simulink model "heaveCompMichael_v03_tollax_spesial"  (R2021b)
settings: Solver=VariableStepAuto  StartTime=0.0  StopTime=50  RelTol=1e-3
model workspace (MATLAB code in the model file):
  | %fluid data
  | rho = 875;
  | %valve config
  | P_r = 70e5;
  | Cd = 0.7;
  | Q_r = 200/6e4;
  | AdMax = Q_r/Cd/sqrt(2/rho*P_r/2);
  | 
  | g = 9.81;                   %gravity
  | zw = 0.8;                   %wave amplitude
  | tw = 10;                    %total wave period
  | ig = 46;                    %gear ratio gearbox
  | m = 9000;                   %mass of payload
  | mueq = 0.15;                %friction coeffisient
  | dd = 0.45;                  %diameter drum
  | nyv = 0.92;                 %volumetric effissiency
  | rd = dd/2;                  %radius drum
  | omega0 = 5;                 %velosity in friction equation
  | omegap = 1500;              %velosity hpu pump
  | nsh = 3;
  | gearrationsh = nsh.*2;
libraries: fl_lib x18, nesl_utility x11, sh_lib x4, slpidlib x1
settings Model: Creator=tolla  LastModifiedBy=marcu

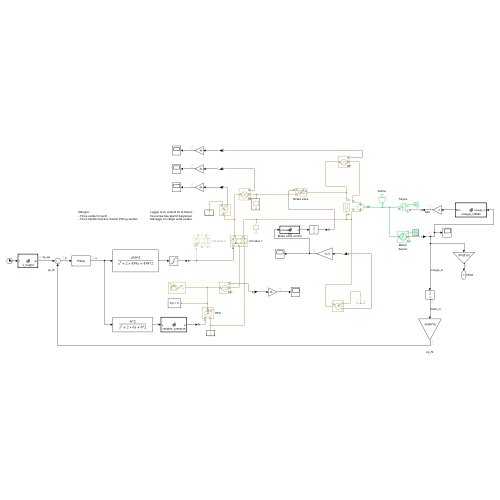
[thumbnail: Simulink's stored preview of the top-level diagram]
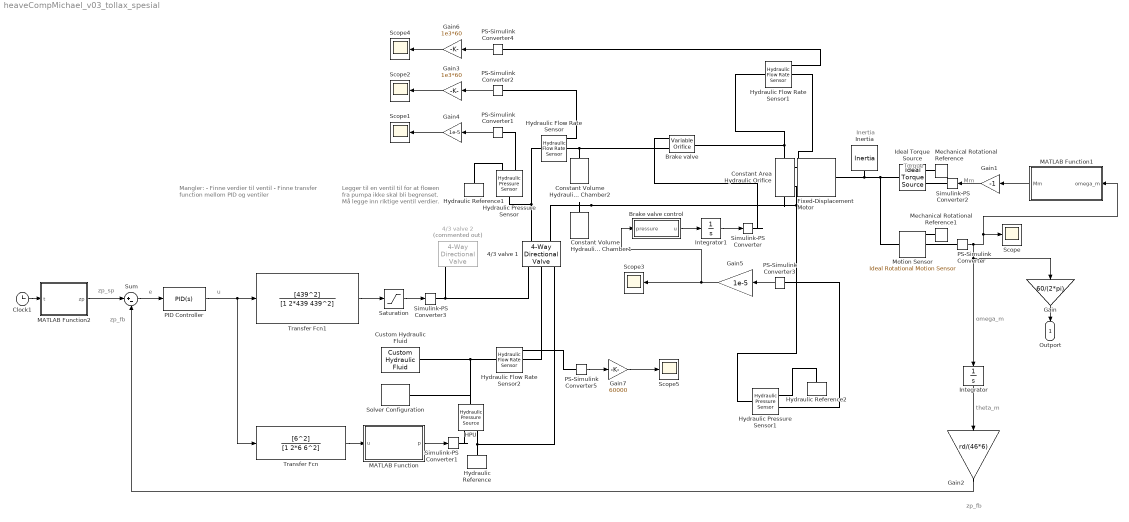
== system heaveCompMichael_v03_tollax_spesial ==
  note: Mangler:
      | - Finne verdier til ventil
      | - Finne transfer function mellom PID og ventiler
  note: Mm
  note: Legger til en ventil til for at flowen
      | fra pumpa ikke skal bli begrenset.
      | Må legge inn riktige ventil verdier.
  note: e
  note: u
  note: zp_fb
  note: zp_sp
  note: zp_fb
  note: theta_m
  note: omega_m
  note: Torque
  note: Inertia
  4/3 valve 1 : sh_lib/Valves/Directional Valves/4-Way Directional Valve  area_spec=sh.valves.directional_valves.enum.area_spec.identical  mdl_type_identical=sh.valves.directional_valves.enum.mdl_type.linear  mdl_type_different=sh.valves.directional_valves.enum.mdl_type.linear  interp_method_identical=sh.valves.directional_valves.enum.interp_method.linear  interp_method_different=sh.valves.directional_valves.enum.interp_method.linear  extrap_method_identical=sh.valves.directional_valves.enum.extrap_method.linear  extrap_method_different=sh.valves.directional_valves.enum.extrap_method.linear  A_leak=1e-12 m^2  C_d=Cd  lam_spec=sh.valves.directional_valves.enum.lam_spec.pressure_ratio  B_lam=0.999  Re_cr=12  opening_max=1 m  area_max=3.7646e-5 m^2  opening_max_P_A=0.005 m  area_max_P_A=0.5e-4 m^2  opening_max_P_B=0.005 m  area_max_P_B=0.5e-4 m^2  opening_max_A_T=0.005 m  area_max_A_T=0.5e-4 m^2  opening_max_B_T=0.005 m  area_max_B_T=0.5e-4 m^2  opening_area_tab=[-.002, 0, .002, .005, .015] m  area_tab=[1e-09, 2.0352e-07, 4.0736e-05, .00011438, .00034356] m^2  opening_flow_rate_tab=[-.002, 0, .002, .005, .015] m  pressure_tab=[-10000000, -5000000, -2000000, 2000000, 5000000, 10000000] Pa  flow_rate_tab=[-1e-07, -7.0711e-08, -4.4721e-08, 4.4721e-08, 7.0711e-08, 1e-07; -2.0352e-05, -1.4391e-05, -9.1017e-06, 9.1017e-06, 1.4391e-05, 2.0352e-05; -.0040736, -.0028805, -.0018218, .0018218, .0028805, .0040736; -.011438, -.0080879, -.0051152, .0051152, .0080879, .011438; -.034356, -.024293, -.015364, .015364, .024293, .034356] m^3/s  opening_area_tab_P_A=[-.002, 0, .002, .005, .015] m  area_tab_P_A=[1e-09, 2.0352e-07, 4.0736e-05, .00011438, .00034356] m^2  opening_flow_rate_tab_P_A=[-.002, 0, .002, .005, .015] m  pressure_tab_P_A=[-10000000, -5000000, -2000000, 2000000, 5000000, 10000000] Pa  flow_rate_tab_P_A=[-1e-07, -7.0711e-08, -4.4721e-08, 4.4721e-08, 7.0711e-08, 1e-07; -2.0352e-05, -1.4391e-05, -9.1017e-06, 9.1017e-06, 1.4391e-05, 2.0352e-05; -.0040736, -.0028805, -.0018218, .0018218, .0028805, .0040736; -.011438, -.0080879, -.0051152, .0051152, .0080879, .011438; -.034356, -.024293, -.015364, .015364, .024293, .034356] m^3/s  opening_area_tab_P_B=[-.002, 0, .002, .005, .015] m  area_tab_P_B=[1e-09, 2.0352e-07, 4.0736e-05, .00011438, .00034356] m^2  opening_flow_rate_tab_P_B=[-.002, 0, .002, .005, .015] m  pressure_tab_P_B=[-10000000, -5000000, -2000000, 2000000, 5000000, 10000000] Pa  flow_rate_tab_P_B=[-1e-07, -7.0711e-08, -4.4721e-08, 4.4721e-08, 7.0711e-08, 1e-07; -2.0352e-05, -1.4391e-05, -9.1017e-06, 9.1017e-06, 1.4391e-05, 2.0352e-05; -.0040736, -.0028805, -.0018218, .0018218, .0028805, .0040736; -.011438, -.0080879, -.0051152, .0051152, .0080879, .011438; -.034356, -.024293, -.015364, .015364, .024293, .034356] m^3/s  opening_area_tab_A_T=[-.002, 0, .002, .005, .015] m  area_tab_A_T=[1e-09, 2.0352e-07, 4.0736e-05, .00011438, .00034356] m^2  opening_flow_rate_tab_A_T=[-.002, 0, .002, .005, .015] m  pressure_tab_A_T=[-10000000, -5000000, -2000000, 2000000, 5000000, 10000000] Pa  flow_rate_tab_A_T=[-1e-07, -7.0711e-08, -4.4721e-08, 4.4721e-08, 7.0711e-08, 1e-07; -2.0352e-05, -1.4391e-05, -9.1017e-06, 9.1017e-06, 1.4391e-05, 2.0352e-05; -.0040736, -.0028805, -.0018218, .0018218, .0028805, .0040736; -.011438, -.0080879, -.0051152, .0051152, .0080879, .011438; -.034356, -.024293, -.015364, .015364, .024293, .034356] m^3/s  opening_area_tab_B_T=[-.002, 0, .002, .005, .015] m  area_tab_B_T=[1e-09, 2.0352e-07, 4.0736e-05, .00011438, .00034356] m^2  opening_flow_rate_tab_B_T=[-.002, 0, .002, .005, .015] m  pressure_tab_B_T=[-10000000, -5000000, -2000000, 2000000, 5000000, 10000000] Pa  flow_rate_tab_B_T=[-1e-07, -7.0711e-08, -4.4721e-08, 4.4721e-08, 7.0711e-08, 1e-07; -2.0352e-05, -1.4391e-05, -9.1017e-06, 9.1017e-06, 1.4391e-05, 2.0352e-05; -.0040736, -.0028805, -.0018218, .0018218, .0028805, .0040736; -.011438, -.0080879, -.0051152, .0051152, .0080879, .011438; -.034356, -.024293, -.015364, .015364, .024293, .034356] m^3/s  x_0_P_A=0 m  x_0_P_B=0 m  x_0_A_T=0 m  x_0_B_T=0 m
      settings: InternalSimscapePortConfiguration="{\"Bottom\":[],\"Left\":[{\"id\":\"A\",\"label\":\"A\",\"type\":\"foundation.hydraulic.hydraulic\"},{\"id\":\"B\",\"label\":\"B\",\"type\":\"foundation.hydraulic.hydraulic\"}],\"Right\":[{\"id\":\"S\",\"label\":\"S\",\"type\":\"input\"},{\"id\":\"P\",\"label\":\"P\",\"type\":\"foundation.hydraulic.hydraulic\"},{\"id\":\"T\",\"label\":\"T\",\"type\":\"foundation.hydraulic.hydraulic\"}],\"Top\":[]}"
  4/3 valve 2 : sh_lib/Valves/Directional Valves/4-Way Directional Valve  Commented=on  area_spec=sh.valves.directional_valves.enum.area_spec.identical  mdl_type_identical=sh.valves.directional_valves.enum.mdl_type.linear  mdl_type_different=sh.valves.directional_valves.enum.mdl_type.linear  interp_method_identical=sh.valves.directional_valves.enum.interp_method.linear  interp_method_different=sh.valves.directional_valves.enum.interp_method.linear  extrap_method_identical=sh.valves.directional_valves.enum.extrap_method.linear  extrap_method_different=sh.valves.directional_valves.enum.extrap_method.linear  A_leak=1e-12 m^2  C_d=Cd  lam_spec=sh.valves.directional_valves.enum.lam_spec.pressure_ratio  B_lam=0.999  Re_cr=12  opening_max=1 m  area_max=3.7646e-5 m^2  opening_max_P_A=0.005 m  area_max_P_A=0.5e-4 m^2  opening_max_P_B=0.005 m  area_max_P_B=0.5e-4 m^2  opening_max_A_T=0.005 m  area_max_A_T=0.5e-4 m^2  opening_max_B_T=0.005 m  area_max_B_T=0.5e-4 m^2  opening_area_tab=[-.002, 0, .002, .005, .015] m  area_tab=[1e-09, 2.0352e-07, 4.0736e-05, .00011438, .00034356] m^2  opening_flow_rate_tab=[-.002, 0, .002, .005, .015] m  pressure_tab=[-10000000, -5000000, -2000000, 2000000, 5000000, 10000000] Pa  flow_rate_tab=[-1e-07, -7.0711e-08, -4.4721e-08, 4.4721e-08, 7.0711e-08, 1e-07; -2.0352e-05, -1.4391e-05, -9.1017e-06, 9.1017e-06, 1.4391e-05, 2.0352e-05; -.0040736, -.0028805, -.0018218, .0018218, .0028805, .0040736; -.011438, -.0080879, -.0051152, .0051152, .0080879, .011438; -.034356, -.024293, -.015364, .015364, .024293, .034356] m^3/s  opening_area_tab_P_A=[-.002, 0, .002, .005, .015] m  area_tab_P_A=[1e-09, 2.0352e-07, 4.0736e-05, .00011438, .00034356] m^2  opening_flow_rate_tab_P_A=[-.002, 0, .002, .005, .015] m  pressure_tab_P_A=[-10000000, -5000000, -2000000, 2000000, 5000000, 10000000] Pa  flow_rate_tab_P_A=[-1e-07, -7.0711e-08, -4.4721e-08, 4.4721e-08, 7.0711e-08, 1e-07; -2.0352e-05, -1.4391e-05, -9.1017e-06, 9.1017e-06, 1.4391e-05, 2.0352e-05; -.0040736, -.0028805, -.0018218, .0018218, .0028805, .0040736; -.011438, -.0080879, -.0051152, .0051152, .0080879, .011438; -.034356, -.024293, -.015364, .015364, .024293, .034356] m^3/s  opening_area_tab_P_B=[-.002, 0, .002, .005, .015] m  area_tab_P_B=[1e-09, 2.0352e-07, 4.0736e-05, .00011438, .00034356] m^2  opening_flow_rate_tab_P_B=[-.002, 0, .002, .005, .015] m  pressure_tab_P_B=[-10000000, -5000000, -2000000, 2000000, 5000000, 10000000] Pa  flow_rate_tab_P_B=[-1e-07, -7.0711e-08, -4.4721e-08, 4.4721e-08, 7.0711e-08, 1e-07; -2.0352e-05, -1.4391e-05, -9.1017e-06, 9.1017e-06, 1.4391e-05, 2.0352e-05; -.0040736, -.0028805, -.0018218, .0018218, .0028805, .0040736; -.011438, -.0080879, -.0051152, .0051152, .0080879, .011438; -.034356, -.024293, -.015364, .015364, .024293, .034356] m^3/s  opening_area_tab_A_T=[-.002, 0, .002, .005, .015] m  area_tab_A_T=[1e-09, 2.0352e-07, 4.0736e-05, .00011438, .00034356] m^2  opening_flow_rate_tab_A_T=[-.002, 0, .002, .005, .015] m  pressure_tab_A_T=[-10000000, -5000000, -2000000, 2000000, 5000000, 10000000] Pa  flow_rate_tab_A_T=[-1e-07, -7.0711e-08, -4.4721e-08, 4.4721e-08, 7.0711e-08, 1e-07; -2.0352e-05, -1.4391e-05, -9.1017e-06, 9.1017e-06, 1.4391e-05, 2.0352e-05; -.0040736, -.0028805, -.0018218, .0018218, .0028805, .0040736; -.011438, -.0080879, -.0051152, .0051152, .0080879, .011438; -.034356, -.024293, -.015364, .015364, .024293, .034356] m^3/s  opening_area_tab_B_T=[-.002, 0, .002, .005, .015] m  area_tab_B_T=[1e-09, 2.0352e-07, 4.0736e-05, .00011438, .00034356] m^2  opening_flow_rate_tab_B_T=[-.002, 0, .002, .005, .015] m  pressure_tab_B_T=[-10000000, -5000000, -2000000, 2000000, 5000000, 10000000] Pa  flow_rate_tab_B_T=[-1e-07, -7.0711e-08, -4.4721e-08, 4.4721e-08, 7.0711e-08, 1e-07; -2.0352e-05, -1.4391e-05, -9.1017e-06, 9.1017e-06, 1.4391e-05, 2.0352e-05; -.0040736, -.0028805, -.0018218, .0018218, .0028805, .0040736; -.011438, -.0080879, -.0051152, .0051152, .0080879, .011438; -.034356, -.024293, -.015364, .015364, .024293, .034356] m^3/s  x_0_P_A=0 m  x_0_P_B=0 m  x_0_A_T=0 m  x_0_B_T=0 m
      settings: InternalSimscapePortConfiguration="{\"Bottom\":[],\"Left\":[{\"id\":\"A\",\"label\":\"A\",\"type\":\"foundation.hydraulic.hydraulic\"},{\"id\":\"B\",\"label\":\"B\",\"type\":\"foundation.hydraulic.hydraulic\"}],\"Right\":[{\"id\":\"S\",\"label\":\"S\",\"type\":\"input\"},{\"id\":\"P\",\"label\":\"P\",\"type\":\"foundation.hydraulic.hydraulic\"},{\"id\":\"T\",\"label\":\"T\",\"type\":\"foundation.hydraulic.hydraulic\"}],\"Top\":[]}"
  Brake valve : sh_lib/Orifices/Variable Orifice  mdl_type=1  area_max=1.2677e-4 m^2  opening_max=1 m  opening_tab=[-.002, 0, .002, .005, .015] m  area_tab=[1e-09, 2.0352e-07, 4.0736e-05, .00011438, .00034356] m^2  pressure_tab=[-10000000, -5000000, -2000000, 2000000, 5000000, 10000000] Pa  flow_rate_tab=[-1e-07, -7.0711e-08, -4.4721e-08, 4.4721e-08, 7.0711e-08, 1e-07; -2.0352e-05, -1.4391e-05, -9.1017e-06, 9.1017e-06, 1.4391e-05, 2.0352e-05; -.0040736, -.0028805, -.0018218, .0018218, .0028805, .0040736; -.011438, -.0080879, -.0051152, .0051152, .0080879, .011438; -.034356, -.024293, -.015364, .015364, .024293, .034356] m^3/s  interp_method=1  extrap_method=1  or=1  C_d=0.7  x_0=1 m  A_leak=1e-12 m^2  lam_spec=1  B_lam=0.999  Re_cr=12  flow_rate_specify=off  flow_rate_priority=None  flow_rate=0 m^3/s  flow_rate_nominal_specify=off  flow_rate_nominal_unit=m^3/s  flow_rate_nominal_value=1  pressure_drop_specify=off  pressure_drop_priority=None  pressure_drop=0 Pa  pressure_drop_nominal_specify=off  pressure_drop_nominal_unit=Pa  pressure_drop_nominal_value=1
      settings: InternalSimscapePortConfiguration="{\"Bottom\":[],\"Left\":[{\"id\":\"S\",\"label\":\"S\",\"type\":\"input\"},{\"id\":\"A\",\"label\":\"A\",\"type\":\"foundation.hydraulic.hydraulic\"}],\"Right\":[{\"id\":\"B\",\"label\":\"B\",\"type\":\"foundation.hydraulic.hydraulic\"}],\"Top\":[]}"
  Brake valve control : MATLAB Function  TreatAsAtomicUnit=on
  Clock1 : Clock
  Constant Area Hydraulic Orifice : fl_lib/Hydraulic/Hydraulic Elements/Constant Area Hydraulic Orifice  area=1e-12 m^2  C_d=0.7  lam_spec=1  B_lam=0.999  Re_cr=12  q_specify=off  q_priority=None  q=1e-3 m^3/s  q_nominal_specify=off  q_nominal_unit=m^3/s  q_nominal_value=1  p_specify=off  p_priority=None  p=0 Pa  p_nominal_specify=off  p_nominal_unit=Pa  p_nominal_value=1
      settings: InternalSimscapePortConfiguration="{\"Bottom\":[],\"Left\":[{\"id\":\"A\",\"label\":\"A\",\"type\":\"foundation.hydraulic.hydraulic\"}],\"Right\":[{\"id\":\"B\",\"label\":\"B\",\"type\":\"foundation.hydraulic.hydraulic\"}],\"Top\":[]}"
  Constant Volume Hydraulic Chamber1 : fl_lib/Hydraulic/Hydraulic Elements/Constant Volume Hydraulic Chamber  ch_sp=foundation.enum.chamberGeometry.volume  wall_type=foundation.enum.chamber_spec.rigid  ch_volume=0.5e-3 m^3  d_in=1e-2 m  length=1 m  pr_r_coef=1.2e-12 m/Pa  time_const=0.01 s  k_sh=1.4  pressure_specify=off  pressure_priority=High  pressure=0 Pa  pressure_nominal_specify=off  pressure_nominal_unit=Pa  pressure_nominal_value=1  diameter_incr_specify=off  diameter_incr_priority=High  diameter_incr=0 m  diameter_incr_nominal_specify=off  diameter_incr_nominal_unit=m  diameter_incr_nominal_value=1  flow_rate_specify=off  flow_rate_priority=None  flow_rate=1e-3 m^3/s  flow_rate_nominal_specify=off  flow_rate_nominal_unit=m^3/s  flow_rate_nominal_value=1
      settings: InternalSimscapePortConfiguration="{\"Bottom\":[],\"Left\":[{\"id\":\"A\",\"label\":\"\",\"type\":\"foundation.hydraulic.hydraulic\"}],\"Right\":[],\"Top\":[]}"
  Constant Volume Hydraulic Chamber2 : fl_lib/Hydraulic/Hydraulic Elements/Constant Volume Hydraulic Chamber  ch_sp=foundation.enum.chamberGeometry.volume  wall_type=foundation.enum.chamber_spec.rigid  ch_volume=0.5e-3 m^3  d_in=1e-2 m  length=1 m  pr_r_coef=1.2e-12 m/Pa  time_const=0.01 s  k_sh=1.4  pressure_specify=off  pressure_priority=High  pressure=0 Pa  pressure_nominal_specify=off  pressure_nominal_unit=Pa  pressure_nominal_value=1  diameter_incr_specify=off  diameter_incr_priority=High  diameter_incr=0 m  diameter_incr_nominal_specify=off  diameter_incr_nominal_unit=m  diameter_incr_nominal_value=1  flow_rate_specify=off  flow_rate_priority=None  flow_rate=1e-3 m^3/s  flow_rate_nominal_specify=off  flow_rate_nominal_unit=m^3/s  flow_rate_nominal_value=1
      settings: InternalSimscapePortConfiguration="{\"Bottom\":[],\"Left\":[{\"id\":\"A\",\"label\":\"\",\"type\":\"foundation.hydraulic.hydraulic\"}],\"Right\":[],\"Top\":[]}"
  Custom Hydraulic Fluid : fl_lib/Hydraulic/Hydraulic Utilities/Custom Hydraulic Fluid  density=875 kg/m^3  viscosity_kin=18e-6 m^2/s  bulk=0.8e9 Pa  alpha=0.005  range_error=2
      settings: InternalSimscapePortConfiguration="{\"Bottom\":[],\"Left\":[],\"Right\":[{\"id\":\"G\",\"label\":\"\",\"type\":\"foundation.hydraulic.hydraulic\"}],\"Top\":[]}"
  Fixed-Displacement Motor : sh_lib/Pumps and Motors/Fixed-Displacement Motor  D=28.1 cm^3/rev  loss_spec=1  w_nominal=616 rad/s  pr_nominal=185 bar  visc_nominal=18 cSt  dens_nominal=rho kg/m^3  efficiency_vol=1  no_load_torque=0 N*m  torque_pressure_coeff=0 N*m/Pa  p_diff_eff_TLU=[100000, 1000000, 2000000] Pa  omega_eff_TLU=[25, 50, 100, 200, 300, 400] rad/s  vol_eff_TLU=[.816, .908, .954, .977, .981, .984; .325, .663, .831, .916, .925, .946; .137, .568, .78, .892, .893, .91]  mech_eff_TLU=[.996, .996, .996, .996, .996, .996; .988, .989, .989, .989, .989, .99; .981, .981, .982, .982, .983, .984]  p_diff_loss_TLU=[100000, 1000000, 2000000] Pa  omega_loss_TLU=[25, 50, 100, 200, 300, 400] rad/s  vol_loss_TLU=[.0282, .0253, .0241, .0235, .0291, .0325; .2596, .1271, .1017, .0917, .1216, .1142; .7874, .1901, .141, .1211, .1797, .1978] * 1e-3 m^3/s  mech_loss_TLU=[.002, .002, .002, .002, .002, .002; .06, .055, .055, .055, .055, .05; .19, .19, .18, .18, .17, .16] N*m  pressure_threshold=1e5 Pa  omega_threshold=10 rad/s  quadrant_check=0  pressure_check=0  min_valid_pressure=0 Pa  vol_eff_min=1e-3  vol_eff_max=1  mech_eff_min=1e-3  mech_eff_max=1
      settings: InternalSimscapePortConfiguration="{\"Bottom\":[],\"Left\":[{\"id\":\"A\",\"label\":\"A\",\"type\":\"foundation.hydraulic.hydraulic\"},{\"id\":\"B\",\"label\":\"B\",\"type\":\"foundation.hydraulic.hydraulic\"}],\"Right\":[{\"id\":\"S\",\"label\":\"S\",\"type\":\"foundation.mechanical.rotational.rotational\"}],\"Top\":[]}"
  Gain : Gain  Gain=60/(2*pi)
  Gain1 : Gain  Gain=-1
  Gain2 : Gain  Gain=rd/(46*6)
  Gain3 : Gain  Gain=1e3*60
  Gain4 : Gain  Gain=1e-5
  Gain5 : Gain  Gain=1e-5
  Gain6 : Gain  Gain=1e3*60
  Gain7 : Gain  Gain=60000
  HPU : fl_lib/Hydraulic/Hydraulic Sources/Hydraulic Pressure Source
      settings: InternalSimscapePortConfiguration="{\"Bottom\":[],\"Left\":[{\"id\":\"P\",\"label\":\"P\",\"type\":\"foundation.hydraulic.hydraulic\"}],\"Right\":[{\"id\":\"S\",\"label\":\"S\",\"type\":\"input\"},{\"id\":\"T\",\"label\":\"T\",\"type\":\"foundation.hydraulic.hydraulic\"}],\"Top\":[]}"
  Hydraulic Flow Rate Sensor : fl_lib/Hydraulic/Hydraulic Sensors/Hydraulic Flow Rate Sensor
  Hydraulic Flow Rate Sensor1 : fl_lib/Hydraulic/Hydraulic Sensors/Hydraulic Flow Rate Sensor
  Hydraulic Flow Rate Sensor2 : fl_lib/Hydraulic/Hydraulic Sensors/Hydraulic Flow Rate Sensor
  Hydraulic Pressure Sensor : fl_lib/Hydraulic/Hydraulic Sensors/Hydraulic Pressure Sensor
  Hydraulic Pressure Sensor1 : fl_lib/Hydraulic/Hydraulic Sensors/Hydraulic Pressure Sensor
  Hydraulic Reference : fl_lib/Hydraulic/Hydraulic Elements/Hydraulic Reference
  Hydraulic Reference1 : fl_lib/Hydraulic/Hydraulic Elements/Hydraulic Reference
  Hydraulic Reference2 : fl_lib/Hydraulic/Hydraulic Elements/Hydraulic Reference
  Ideal Torque Source : fl_lib/Mechanical/Mechanical Sources/Ideal Torque Source
  Inertia : fl_lib/Mechanical/Rotational Elements/Inertia  Tag=Factory Generic  inertia=0.0072 kg*m^2  num_ports=foundation.enum.numPorts2.one  w_specify=off  w_priority=High  w=0 rad/s  w_nominal_specify=off  w_nominal_unit=rad/s  w_nominal_value=1  t_specify=off  t_priority=High  t=0 N*m  t_nominal_specify=off  t_nominal_unit=N*m  t_nominal_value=1
  Integrator : Integrator
  Integrator1 : Integrator
  MATLAB Function : MATLAB Function  TreatAsAtomicUnit=on
  MATLAB Function1 : MATLAB Function  TreatAsAtomicUnit=on
  MATLAB Function2 : MATLAB Function  TreatAsAtomicUnit=on
  Mechanical Rotational Reference : fl_lib/Mechanical/Rotational Elements/Mechanical Rotational Reference
  Mechanical Rotational Reference1 : fl_lib/Mechanical/Rotational Elements/Mechanical Rotational Reference
  Motion Sensor : fl_lib/Mechanical/Mechanical Sensors/Ideal Rotational Motion Sensor  Tag=Factory Generic  reference=foundation.enum.MeasurementReference.difference  acceleration_port=false  velocity_port=true  position_port=true  wrap_angle=simscape.enum.onoff.on  offset=0 rad
  PID Controller : slpidlib/PID Controller  Controller=PID  Form=Parallel  TimeDomain=Continuous-time  UseExternalTs=off  SampleTime=-1  IntegratorMethod=Forward Euler  FilterMethod=Forward Euler  ControllerParametersSource=internal  P=20  I=0  D=0  N=100  UseFilter=on  TunerSelectOption=Transfer Function Based (PID Tuner App)  InitialConditionSource=internal  InitialConditionForIntegrator=0  InitialConditionForFilter=0  DifferentiatorICPrevScaledInput=0  ExternalReset=none  TrackingMode=off  Kt=1  LimitOutput=off  SatLimitsSource=internal  UpperSaturationLimit=1  LowerSaturationLimit=-1  LinearizeAsGain=on  AntiWindupMode=none  Kb=1  POutMin=[]  POutMax=[]  IOutMin=[]  IOutMax=[]  DOutMin=[]  DOutMax=[]  NOutMin=[]  NOutMax=[]  SumOutMin=[]  SumOutMax=[]  SaturationOutMin=[]  SaturationOutMax=[]  PParamMin=[]  PParamMax=[]  IParamMin=[]  IParamMax=[]  DParamMin=[]  DParamMax=[]  NParamMin=[]  NParamMax=[]  KbParamMin=[]  KbParamMax=[]  KtParamMin=[]  KtParamMax=[]  KbOutMin=[]  KbOutMax=[]  KtOutMin=[]  KtOutMax=[]  IntegratorOutMin=[]  IntegratorOutMax=[]  FilterOutMin=[]  FilterOutMax=[]  SumI1OutMin=[]  SumI1OutMax=[]  SumI2OutMin=[]  SumI2OutMax=[]  SumI3OutMin=[]  SumI3OutMax=[]  SumI4OutMin=[]  SumI4OutMax=[]  SumDOutMin=[]  SumDOutMax=[]  DifferentiatorOutMin=[]  DifferentiatorOutMax=[]  FilterDiffOutCoefMin=[]  FilterDiffOutCoefMax=[]  ReciprocalOutMin=[]  ReciprocalOutMax=[]  SumDenOutMin=[]  SumDenOutMax=[]  SumNumOutMin=[]  SumNumOutMax=[]  DivideOutMin=[]  DivideOutMax=[]  UdiffTsProdOutMin=[]  UdiffTsProdOutMax=[]  NTsProdOutMin=[]  NTsProdOutMax=[]  UintegralTsProdOutMin=[]  UintegralTsProdOutMax=[]  UngainTsProdOutMin=[]  UngainTsProdOutMax=[]  IntegratorContinuousStateAttributes=''  IntegratorStateMustResolveToSignalObject=off  IntegratorRTWStateStorageClass=Auto  FilterContinuousStateAttributes=''  FilterStateMustResolveToSignalObject=off  FilterRTWStateStorageClass=Auto  ParallelPVariant=InternalParameters  IdealPVariant=Disabled  IVariant=InternalParameters  DVariant=InternalParameters  IntegratorVariant=Continuous  SatVariant=Disabled  AWVariant=Passthrough  PCopyVariant=Disabled  TRVariant=Disabled  FdbkBlocksVariant=Forward  IdealPFdbkVariant=Disabled  SatFdbkVariant=Disabled  DerivativeFilterVariant=ContFilter  NVariant=InternalParameters  NCopyVariant=Disabled  FilterICVariant=InternalICsFilter  IntegratorICVariant=InternalICs  ExternalResetVariant=Disabled  TRSumVariant=Passthrough  SumFdbkVariant=Disabled  SumVariant=Sum_PID  TsampFilterVariant=InternalTs  TsampNgainVariant=Passthrough  TsampIntegralVariant=Passthrough  ExternalSaturationOutDataTypeStr=Inherit: Same as second input
  PS-Simulink Converter{,1..5} (6 alike) : nesl_utility/PS-Simulink Converter  PhysicalDomain=network_engine_domain  SubClassName=ps_output  LeftPortType=input  RightPortType=output  PseudoPeriodic=off  Frequencies=[]  VectorFormat=inherit  Unit=inherit  AffineConversion=off
  Saturation : Saturate  UpperLimit=1  LowerLimit=-1
  Scope{,1..5} (6 alike) : Scope
  Simulink-PS Converter{,1..3} (4 alike) : nesl_utility/Simulink-PS Converter  PhysicalDomain=network_engine_domain  SubClassName=ps_input  LeftPortType=input  RightPortType=output  PseudoPeriodic=off  Frequencies=[]  NoiseDistribution=none  NoiseParameters=[]  Unit=1  AffineConversion=off  FilteringAndDerivatives=provide  SimscapeFilterOrder=1  InputFilterTimeConstant=0.001  UdotUserProvided=0
  Solver Configuration : nesl_utility/Solver Configuration  PhysicalDomain=network_engine_domain  SubClassName=solver  LeftPortType=input  RightPortType=generic  Tones=[]  Harmonics=[]  SimulateNoise=off  Profile=off  UseLocalSampling=off  EnableSwitchedLinearOptims=on  FrequencyDomain=off  UseCCode=off  RelTol=0.001  AbsTol=1e-06  MinStep=1e-09  ToWorkspace=off  RevertToSquareIcSolve=off  NumHomotopyIterations=100  PhasorMode=off  PhasorModeNumHarmonics=1  ConsistencySolver=NEWTON_FTOL  IndexReductionMethod=DerivativeReplacement  DoDC=off  ResidualTolerance=1e-09  ConsistencyTolSource=GLOBAL  ConsistencyAbsTol=0.001  ConsistencyRelTol=0.001  ConsistencyTolFactor=0.001  UseLocalSolver=off  LocalSolverChoice=NE_BACKWARD_EULER_ADVANCER  ResolveIndetEquations=on  FunctionEvalNumThread=1  LocalSolverSampleTime=0.001  DoFixedCost=off  MaxNonlinIter=3  MaxModeIter=2  ComputeImpulses=off  ImpulseIterations=2  LinearAlgebra=auto  LinearAlgebraNumThread=0  EquationFormulation=NE_TIME_EF  DelaysMemoryBudget=1024  AutomaticFiltering=on  FilteringTimeConstant=0.001  PartitionStorageMethod=AS_NEEDED  PartitionMemoryBudget=1024  PartitionMethod=ROBUST
  Sum : Sum  Inputs=|+-
  Transfer Fcn : TransferFcn  Numerator=[6^2]  Denominator=[1 2*6 6^2]
  Transfer Fcn1 : TransferFcn  Numerator=[439^2]  Denominator=[1 2*439 439^2]
  Outport : Outport  SignalName=RPM
  wires:
  MATLAB Function1/1(Mm) -> Gain1/1
  PS-Simulink Converter/1 -> Integrator/1, Gain/1, MATLAB Function1/1(omega_m), Scope/1
  Gain1/1 -> Simulink-PS Converter2/1
  Gain/1 -> Outport/1
  Clock1/1 -> MATLAB Function2/1(t)
  MATLAB Function2/1(zp) -> Sum/1
  Sum/1 -> PID Controller/1
  Integrator/1 -> Gain2/1
  Gain2/1 -> Sum/2
  PS-Simulink Converter1/1 -> Gain4/1
  PS-Simulink Converter2/1 -> Gain3/1
  Gain3/1 -> Scope2/1
  Gain4/1 -> Scope1/1
  PS-Simulink Converter3/1 -> Gain5/1
  Gain5/1 -> Brake valve control/1(pressure), Scope3/1
  Integrator1/1 -> Simulink-PS Converter/1
  Brake valve control/1(u) -> Integrator1/1
  PS-Simulink Converter4/1 -> Gain6/1
  Gain6/1 -> Scope4/1
  Saturation/1 -> Simulink-PS Converter3/1
  PID Controller/1 -> Transfer Fcn/1, Transfer Fcn1/1
  Transfer Fcn1/1 -> Saturation/1
  Transfer Fcn/1 -> MATLAB Function/1(u)
  MATLAB Function/1(p) -> Simulink-PS Converter1/1
  Gain7/1 -> Scope5/1
  PS-Simulink Converter5/1 -> Gain7/1
  connections:
  HPU/RConn2 -- 4/3 valve 1/RConn3 -- Hydraulic Reference/LConn1
  Solver Configuration/RConn1 -- HPU/LConn1 -- Custom Hydraulic Fluid/RConn1 -- Hydraulic Flow Rate Sensor2/LConn1
  Hydraulic Pressure Sensor1/LConn1 -- Constant Volume Hydraulic Chamber1/LConn1 -- 4/3 valve 1/LConn2 -- Constant Area Hydraulic Orifice/RConn1 -- Fixed-Displacement Motor/LConn2
  4/3 valve 1/LConn1 -- Hydraulic Pressure Sensor/LConn1 -- Hydraulic Flow Rate Sensor/LConn1
  4/3 valve 1/RConn1 -- 4/3 valve 2/RConn1 -- Simulink-PS Converter3/RConn1
  Simulink-PS Converter1/RConn1 -- HPU/RConn1
  Fixed-Displacement Motor/RConn1 -- Inertia/LConn1 -- Motion Sensor/LConn1 -- Ideal Torque Source/LConn1
  Simulink-PS Converter2/RConn1 -- Ideal Torque Source/RConn1
  Mechanical Rotational Reference/LConn1 -- Ideal Torque Source/RConn2
  Motion Sensor/RConn2 -- PS-Simulink Converter/LConn1
  Mechanical Rotational Reference1/LConn1 -- Motion Sensor/RConn1
  Hydraulic Pressure Sensor/RConn2 -- PS-Simulink Converter1/LConn1
  Hydraulic Reference1/LConn1 -- Hydraulic Pressure Sensor/RConn1
  Constant Volume Hydraulic Chamber2/LConn1 -- Brake valve/LConn2 -- Hydraulic Flow Rate Sensor/RConn2
  PS-Simulink Converter2/LConn1 -- Hydraulic Flow Rate Sensor/RConn1
  Hydraulic Reference2/LConn1 -- Hydraulic Pressure Sensor1/RConn1
  Hydraulic Pressure Sensor1/RConn2 -- PS-Simulink Converter3/LConn1
  PS-Simulink Converter4/LConn1 -- Hydraulic Flow Rate Sensor1/RConn1
  Fixed-Displacement Motor/LConn1 -- Hydraulic Flow Rate Sensor1/RConn2
  Constant Area Hydraulic Orifice/LConn1 -- Brake valve/RConn1 -- Hydraulic Flow Rate Sensor1/LConn1
  Simulink-PS Converter/RConn1 -- Brake valve/LConn1
  Hydraulic Flow Rate Sensor2/RConn2 -- 4/3 valve 1/RConn2
  Hydraulic Flow Rate Sensor2/RConn1 -- PS-Simulink Converter5/LConn1

== matlab function heaveCompMichael_v03_tollax_spesial/Brake valve control ==
  data: pressure input; u output
function u = fcn(pressure)

p_cr = 20; % bar
dp_fo = 10; % bar, delta p_fully_open

u = (pressure-p_cr)/dp_fo;

if(u >= 1)
    u = 1;
elseif(u < 0)
    u = 0;
end

== matlab function heaveCompMichael_v03_tollax_spesial/MATLAB Function2 ==
  data: t input; zp output
function zp = z_height(t)

z_w = 0.8; % m
T_w = 10; % s

zp = z_w * sin((2*pi*t)/T_w);

== matlab function heaveCompMichael_v03_tollax_spesial/MATLAB Function ==
  data: u input; p output
function p = variable_pressure(u)

if(u > 0)
    p = 225e5; % Pa
else
    p = 40e5; % Pa
end

== matlab function heaveCompMichael_v03_tollax_spesial/MATLAB Function1 ==
  data: omega_m input; Mm output
function Mm = omega_m2Mm(omega_m)

n_sh = 3; % -
i_g = 46; % -
m_pl = 9000; % kg
d_D = 0.45; % m
mu_eq = 0.15; % -
omega_0 = 5; % rad/s
g = 9.81; % m/(s*s)

Mm = (m_pl*g*d_D)/(2*n_sh*2*i_g) * (1 + mu_eq * tanh(omega_m/omega_0));
